simulink model "a2bcpwm_inverter_final"  (R2021b)
settings: Solver=VariableStepAuto  StartTime=0.0  StopTime=1.8  RelTol=1e-3
libraries: spsMosfetLib x8, spsSeriesRLCBranchLib x6, spsVoltageMeasurementLib x5, spsCurrentMeasurementLib x3, spsRMSLib x3, spsFourierLib x2, spsTriangleGeneratorLib x2, spsDCVoltageSourceLib x1, spsDiodeLib x1, spsMeanLib x1, spspowerguiLib x1
settings Model: Creator=adars  LastModifiedBy=basti
settings SolverCC: ZeroCrossAlgorithm=Adaptive
settings DebuggingCC: IgnoredZcDiagnostic=none  UnconnectedInputMsg=none  UnconnectedOutputMsg=none  UnconnectedLineMsg=none
settings ModelReferenceCC: EnableRefExpFcnMdlSchedulingChecks=off
settings RTWCC: DLArmComputeVersion=20.02.1

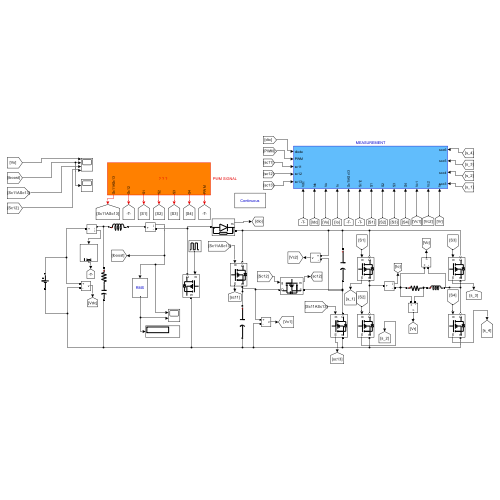
[thumbnail: Simulink's stored preview of the top-level diagram]
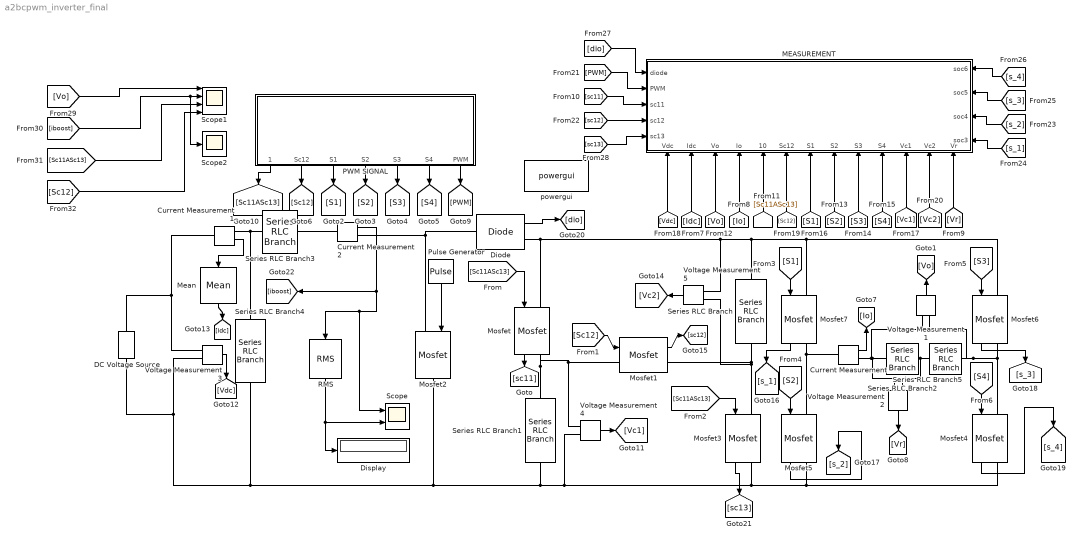
== system a2bcpwm_inverter_final ==
  Current Measurement : spsCurrentMeasurementLib/Current Measurement  PhasorSimulation=off  OutputType=Complex  PSBequivalent=0
  Current Measurement1 : spsCurrentMeasurementLib/Current Measurement  PhasorSimulation=off  OutputType=Complex  PSBequivalent=0
  Current Measurement2 : spsCurrentMeasurementLib/Current Measurement  PhasorSimulation=off  OutputType=Complex  PSBequivalent=0
  DC Voltage Source : spsDCVoltageSourceLib/DC Voltage Source  Amplitude=24  Measurements=None
  Diode : spsDiodeLib/Diode  Ron=0.001  Lon=0  Vf=0.8  IC=0  UseSnubber=0  Rs=500  Cs=250e-9  Measurements=on
  Display : Display
  MEASUREMENT : Subsystem
      settings: PortSchema="{\"entries\":[{\"content\":{\"sides\":[{\"content\":{\"connectorIds\":[\"In1\",\"In2\",\"In3\",\"In4\",\"In5\"]},\"type\":\"ConnectorPlacement.EquallySpacedRectSide\",\"uuid\":\"d6dfc44f-8fba-4c4a-86af-0984d0d1ef13\"},{\"content\":{\"connectorIds\":[\"In19\",\"In20\",\"In21\",\"In22\"],\"side\":\"RIGHT\"},\"type\":\"ConnectorPlacement.EquallySpacedRectSide\",\"uuid\":\"d6149925-38bb-4c16-a1b8-fa53fbdb5b8e\"},{\"content\":{\"connectorIds\":[],\"side\":\"TOP\"},\"type\":\"ConnectorPlacement.EquallySpacedRectSide\",\"uuid\":\"0a993214-5764-4564-a5db-9fa5a3117433\"},{\"content\":{\"connectorIds\":[\"In6\",\"In7\",\"In8\",\"In9\",\"In10\",\"In11\",\"In12\",\"In13\",\"In14\",\"In15\",\"In16\",\"In17\",\"In18\"],\"side\":\"BOTTOM\"},\"type\":\"ConnectorPlacement.EquallySpacedRectSide\",\"uuid\":\"ef2b73df-4ab0-44d0-8380-8491338002fd\"}]},\"type\":\"ConnectorPlacement.EquallySpacedConnector\",\"uuid\":\"c728dddf-1d1a-4ffc-a551-ed9f27d05892\"}],\"packageUris\":[\"http://schema.mathworks.com/mf0/Connector/R2020b\"],\"version\":\"1.0\"}"
  Mean : spsMeanLib/Mean  Freq=50  Vinit=0  Ts=0
  Mosfet{,1,3..7} (7 alike) : spsMosfetLib/Mosfet  Ron=0.1  Lon=0  Rd=0.01  Vfd=0  IC=0  Rs=1e5  Cs=inf  Measurements=on
  Mosfet2 : spsMosfetLib/Mosfet  Ron=0.1  Lon=0  Rd=0.01  Vfd=0  IC=0  Rs=1e5  Cs=inf  Measurements=off
  PWM SIGNAL : Subsystem
      mask Display: image('C:\Users\charl\Downloads\Screenshot 2023-01-03 005642.jpg'); % Use "Edit Image" on toolstrip to change.
  Pulse Generator : DiscretePulseGenerator  PulseType=Time based  Period=1/20000  PulseWidth=80
  RMS : spsRMSLib/RMS  TrueRMS=on  Freq=60  RMSInit=120  Ts=0
  Scope : Scope  NumInputPorts=2
  Scope1 : Scope  NumInputPorts=4
  Scope2 : Scope
  Series RLC Branch : spsSeriesRLCBranchLib/Series RLC Branch  LConnTagsString=__new0  RConnTagsString=__new0  BranchType=C  Resistance=1  Inductance=1e-3  SetiL0=off  InitialCurrent=0  Capacitance=3.9e-3  Setx0=off  InitialVoltage=0  Measurements=None
  Series RLC Branch1 : spsSeriesRLCBranchLib/Series RLC Branch  LConnTagsString=__new0  RConnTagsString=__new0  BranchType=C  Resistance=1  Inductance=1e-3  SetiL0=off  InitialCurrent=0  Capacitance=3.9e-3  Setx0=off  InitialVoltage=0  Measurements=None
  Series RLC Branch2 : spsSeriesRLCBranchLib/Series RLC Branch  LConnTagsString=__new0  RConnTagsString=__new0  BranchType=R  Resistance=70  Inductance=150e-3  SetiL0=off  InitialCurrent=0  Capacitance=1e-6  Setx0=off  InitialVoltage=0  Measurements=None
  Series RLC Branch3 : spsSeriesRLCBranchLib/Series RLC Branch  LConnTagsString=__new0  RConnTagsString=__new0  BranchType=L  Resistance=1.5  Inductance=0.9e-3  SetiL0=off  InitialCurrent=0  Capacitance=1e-6  Setx0=off  InitialVoltage=0  Measurements=None
  Series RLC Branch4 : spsSeriesRLCBranchLib/Series RLC Branch  LConnTagsString=__new0  RConnTagsString=__new0  BranchType=RC  Resistance=.0001  Inductance=1e-3  SetiL0=off  InitialCurrent=0  Capacitance=1e-3  Setx0=off  InitialVoltage=0  Measurements=None
  Series RLC Branch5 : spsSeriesRLCBranchLib/Series RLC Branch  LConnTagsString=__new0  RConnTagsString=__new0  BranchType=L  Resistance=100  Inductance=.129  SetiL0=off  InitialCurrent=0  Capacitance=1e-6  Setx0=off  InitialVoltage=0  Measurements=None
  Voltage Measurement{1..5} (5 alike) : spsVoltageMeasurementLib/Voltage Measurement  PhasorSimulation=off  OutputType=Complex  PSBequivalent=0
  powergui : spspowerguiLib/powergui  Priority=1  SimulationMode=Continuous  SampleTime=50e-6  frequency=60  Iterations=50  frequencyindice=0  Pbase=100e6  ErrMax=1e-4  UnitsV=kV  UnitsW=MW  buscounter=0  FunctionMessages=off  echomessages=off  EnableUseOfTLC=off  CurrentSourceSwitches=off  DisableSnubberDevices=off  DisableRonSwitches=off  DisableVfSwitches=off  DisplayEquations=off  AutomaticDiscreteSolvers=off  SolverType=Tustin/Backward Euler (TBE)  Interpol=off  ExternalGateDelay=off  methode=off  Ts=100  x0status=blocks  SPID=on  SwTol=0  HookPort=off  NonlinearTolerance=1e-4  nMaxIteration=100  ContinueOnMaxIteration=off  RestoreLinks=warning  ResistiveCurrentMeasurement=off  Frange=[0:2:500]  Ylog=off  Xlog=on  ShowGrid=off  save=off  variable=ZData  structure=0  ZoomFFT=off  StartTime=0.0  cycles=1  DisplayStyle=1  fundamental=60  FreqAxis=off  MaxFrequency=1000  frequencyindicesteady=1  RmsSteady=1  display=off
  wires:
  PWM SIGNAL/1(Sc11ASc13) -> [Sc11ASc13]
  PWM SIGNAL/6(S4) -> [S4]
  PWM SIGNAL/5(S3) -> [S3]
  PWM SIGNAL/3(S1) -> [S1]
  PWM SIGNAL/2(Sc12) -> [Sc12]
  [Sc11ASc13] -> Mosfet/1
  [Sc12] -> Mosfet1/1
  [Sc11ASc13] -> Mosfet3/1
  [S1] -> Mosfet7/1
  [S2] -> Mosfet5/1
  [S3] -> Mosfet6/1
  [S4] -> Mosfet4/1
  PWM SIGNAL/4(S2) -> [S2]
  Current Measurement/1 -> [Io]
  [Vo] -> MEASUREMENT/8(Vo)
  [Io] -> MEASUREMENT/9(Io)
  [Sc11ASc13] -> MEASUREMENT/10(Sc11ASc13)
  [Sc12] -> MEASUREMENT/11(Sc12)
  [S1] -> MEASUREMENT/12(S1)
  [S2] -> MEASUREMENT/13(S2)
  [S3] -> MEASUREMENT/14(S3)
  [S4] -> MEASUREMENT/15(S4)
  PWM SIGNAL/7(PWM) -> [PWM]
  Pulse Generator/1 -> Mosfet2/1
  Voltage Measurement1/1 -> [Vo]
  [Idc] -> MEASUREMENT/7(Idc)
  Voltage Measurement3/1 -> [Vdc]
  [Vdc] -> MEASUREMENT/6(Vdc)
  Voltage Measurement4/1 -> [Vc1]
  Voltage Measurement5/1 -> [Vc2]
  Current Measurement1/1 -> Mean/1
  Mean/1 -> [Idc]
  [Vc1] -> MEASUREMENT/16(Vc1)
  [Vc2] -> MEASUREMENT/17(Vc2)
  [PWM] -> MEASUREMENT/2(PWM)
  Voltage Measurement2/1 -> [Vr]
  [Vr] -> MEASUREMENT/18(Vr)
  Mosfet/1 -> [sc11]
  Mosfet1/1 -> [sc12]
  [sc12] -> MEASUREMENT/4(sc12)
  [sc11] -> MEASUREMENT/3(sc11)
  Mosfet7/1 -> [s_1]
  Mosfet5/1 -> [s_2]
  Mosfet6/1 -> [s_3]
  Mosfet4/1 -> [s_4]
  [s_2] -> MEASUREMENT/21(soc4)
  [s_1] -> MEASUREMENT/22(soc3)
  [s_3] -> MEASUREMENT/20(soc5)
  [s_4] -> MEASUREMENT/19(soc6)
  Diode/1 -> [dio]
  [dio] -> MEASUREMENT/1(diode)
  Mosfet3/1 -> [sc13]
  [sc13] -> MEASUREMENT/5(sc13)
  Current Measurement2/1 -> [iboost], Scope/1, RMS/1
  RMS/1 -> Display/1, Scope/2
  [Vo] -> Scope1/1
  [iboost] -> Scope2/1, Scope1/2
  [Sc11ASc13] -> Scope1/3
  [Sc12] -> Scope1/4
  connections:
  Mosfet4/LConn1 -- Voltage Measurement1/LConn2 -- Series RLC Branch5/RConn1 -- Mosfet6/RConn1
  Series RLC Branch2/LConn1 -- Current Measurement/RConn1 -- Voltage Measurement1/LConn1 -- Voltage Measurement2/LConn1
  Series RLC Branch/RConn1 -- Mosfet3/LConn1 -- Voltage Measurement5/LConn2 -- Mosfet1/RConn1
  Mosfet/RConn1 -- Voltage Measurement4/LConn1 -- Mosfet1/LConn1 -- Series RLC Branch1/LConn1
  Mosfet7/LConn1 -- Voltage Measurement5/LConn1 -- Mosfet/LConn1 -- Diode/RConn1 -- Series RLC Branch/LConn1 -- Mosfet6/LConn1
  Mosfet7/RConn1 -- Mosfet5/LConn1 -- Current Measurement/LConn1
  Series RLC Branch4/LConn1 -- Current Measurement1/RConn1 -- Series RLC Branch3/LConn1
  Mosfet5/RConn1 -- Voltage Measurement4/LConn2 -- Series RLC Branch1/RConn1 -- DC Voltage Source/LConn1 -- Voltage Measurement3/LConn2 -- Series RLC Branch4/RConn1 -- Mosfet2/RConn1 -- Mosfet3/RConn1 -- Mosfet4/RConn1
  Voltage Measurement3/LConn1 -- DC Voltage Source/RConn1 -- Current Measurement1/LConn1
  Voltage Measurement2/LConn2 -- Series RLC Branch2/RConn1 -- Series RLC Branch5/LConn1
  Mosfet2/LConn1 -- Current Measurement2/RConn1 -- Diode/LConn1
  Current Measurement2/LConn1 -- Series RLC Branch3/RConn1

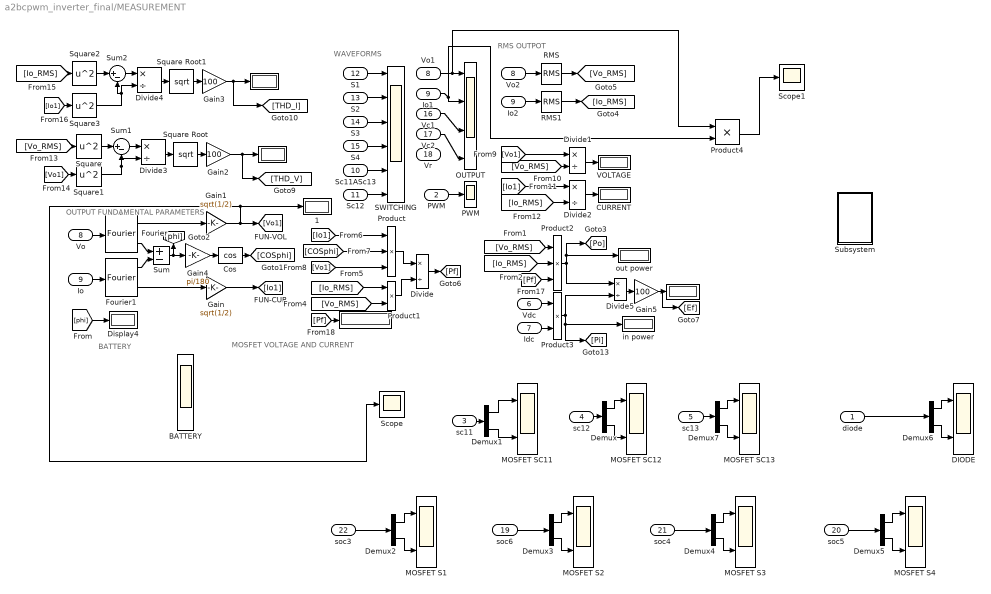
== system a2bcpwm_inverter_final/MEASUREMENT ==
  note: MOSFET VOLTAGE AND
      | CURRENT
  note: BATTERY
  note: WAVEFORMS
  note: OUTPUT FUNDAMENTAL PARAMETERS
  note: RMS OUTPOT
  diode : Inport
  PWM : Inport  Port=2
  sc11 : Inport  Port=3
  sc12 : Inport  Port=4
  sc13 : Inport  Port=5
  Vdc : Inport  Port=6
  Idc : Inport  Port=7
  Vo : Inport  Port=8
  Io : Inport  Port=9
  Sc11ASc13 : Inport  Port=10
  Sc12 : Inport  Port=11
  S1 : Inport  Port=12
  S2 : Inport  Port=13
  S3 : Inport  Port=14
  S4 : Inport  Port=15
  Vc1 : Inport  Port=16
  Vc2 : Inport  Port=17
  Vr : Inport  Port=18
  soc6 : Inport  Port=19
  soc5 : Inport  Port=20
  soc4 : Inport  Port=21
  soc3 : Inport  Port=22
  " " : Display
  "  " : Display
  "   " : Display
  "        " : Display
  "   1" : Display
  "  VOLTAGE  " : Display
  " out power" : Display
  BATTERY : Scope  NumInputPorts=3
  CURRENT : Display
  Cos : Trigonometry  Operator=cos
  DIODE : Scope  NumInputPorts=2
  Demux{,1..7} (8 alike) : Demux  Outputs=2
  Display4 : Display
  Divide{,1..5} (6 alike) : Product  Inputs=*/
  Fourier : spsFourierLib/Fourier  Freq=50  n=1  InInit=[0, 0]  Ts=0
  Fourier1 : spsFourierLib/Fourier  Freq=50  n=1  InInit=[0, 0]  Ts=0
  Gain : Gain  Gain=sqrt(1/2)
  Gain1 : Gain  Gain=sqrt(1/2)
  Gain2 : Gain  Gain=100
  Gain3 : Gain  Gain=100
  Gain4 : Gain  Gain=pi/180
  Gain5 : Gain  Gain=100
  Io1 : InportShadow  Port=9
  Io2 : InportShadow  Port=9
  MOSFET S{1..4} (4 alike) : Scope  NumInputPorts=2
  MOSFET SC11 : Scope  NumInputPorts=2
  MOSFET SC12 : Scope  NumInputPorts=2
  MOSFET SC13 : Scope  NumInputPorts=2
  OUTPUT : Scope  NumInputPorts=4
  "PWM " : Scope
  Product : Product  Inputs=3
  Product1 : Product
  Product2 : Product  Inputs=***
  Product3 : Product  Inputs=**
  Product4 : Product
  RMS : spsRMSLib/RMS  TrueRMS=on  Freq=50  RMSInit=120  Ts=0
  RMS1 : spsRMSLib/RMS  TrueRMS=on  Freq=50  RMSInit=120  Ts=0
  SWITCHING : Scope  NumInputPorts=6
  Scope : Scope
  Scope1 : Scope
  Square{,1..3} (4 alike) : Math  Operator=square  SaturateOnIntegerOverflow=on
  Square Root : Sqrt  SaturateOnIntegerOverflow=on
  Square Root1 : Sqrt  SaturateOnIntegerOverflow=on
  Subsystem : Subsystem
  Sum : Sum  Inputs=+-
  Sum1 : Sum  Inputs=|+-
  Sum2 : Sum  Inputs=|+-
  Vo1 : InportShadow  Port=8
  Vo2 : InportShadow  Port=8
  in power : Display
  wires:
  Sc11ASc13/1 -> SWITCHING/5
  Sc12/1 -> SWITCHING/6
  S1/1 -> SWITCHING/1
  S2/1 -> SWITCHING/2
  S3/1 -> SWITCHING/3
  S4/1 -> SWITCHING/4
  Vo/1 -> Fourier/1
  Io/1 -> Fourier1/1
  Fourier/1 -> Gain1/1
  Fourier/2 -> Sum/1
  Fourier1/1 -> Gain/1
  Fourier1/2 -> Sum/2
  Sum/1 -> Gain4/1, [phi]
  Gain/1 -> [Io1]
  Gain1/1 -> "   1"/1, Scope/1, [Vo1]
  Vo2/1 -> RMS/1
  Io2/1 -> RMS1/1
  RMS1/1 -> [Io_RMS]
  Cos/1 -> [COSphi]
  Product/1 -> Divide/1
  Product1/1 -> Divide/2
  Divide/1 -> [Pf]
  RMS/1 -> [Vo_RMS]
  [Io1] -> Product/1
  [Vo1] -> Product/3
  [COSphi] -> Product/2
  [Io_RMS] -> Product1/1
  [Vo_RMS] -> Product1/2
  [Vo1] -> Divide1/1
  [Vo_RMS] -> Divide1/2
  [Io1] -> Divide2/1
  [Io_RMS] -> Divide2/2
  Divide1/1 -> "  VOLTAGE  "/1
  Divide2/1 -> CURRENT/1
  [Vo_RMS] -> Square/1
  [Vo1] -> Square1/1
  Square/1 -> Sum1/1
  Square1/1 -> Divide3/2, Sum1/2
  Sum1/1 -> Divide3/1
  Divide3/1 -> Square Root/1
  Square2/1 -> Sum2/1
  Sum2/1 -> Divide4/1
  [Io_RMS] -> Square2/1
  [Io1] -> Square3/1
  Square3/1 -> Divide4/2, Sum2/2
  Divide4/1 -> Square Root1/1
  [phi] -> Display4/1
  [Vo_RMS] -> Product2/1
  [Io_RMS] -> Product2/2
  [Pf] -> Product2/3
  Vdc/1 -> Product3/1
  Idc/1 -> Product3/2
  Square Root/1 -> Gain2/1
  Square Root1/1 -> Gain3/1
  Gain4/1 -> Cos/1
  [Pf] -> "        "/1
  Vo1/1 -> Product4/1, OUTPUT/1
  Vc1/1 -> OUTPUT/3
  PWM/1 -> "PWM "/1
  Vc2/1 -> OUTPUT/4
  Io1/1 -> Product4/2, OUTPUT/2
  Divide5/1 -> Gain5/1
  sc12/1 -> Demux/1
  Demux/1 -> MOSFET SC12/1
  Demux/2 -> MOSFET SC12/2
  Demux1/1 -> MOSFET SC11/1
  sc11/1 -> Demux1/1
  Demux1/2 -> MOSFET SC11/2
  Gain2/1 -> "  "/1, [THD_V]
  Gain3/1 -> "   "/1, [THD_I]
  Product3/1 -> [Pi], in power/1, Divide5/2
  Product2/1 -> [Po], " out power"/1, Divide5/1
  Gain5/1 -> [Ef], " "/1
  Demux4/1 -> MOSFET S3/1
  Demux3/2 -> MOSFET S2/2
  soc4/1 -> Demux4/1
  soc6/1 -> Demux3/1
  Demux3/1 -> MOSFET S2/1
  soc5/1 -> Demux5/1
  Demux4/2 -> MOSFET S3/2
  Demux5/1 -> MOSFET S4/1
  Demux5/2 -> MOSFET S4/2
  diode/1 -> Demux6/1
  Demux6/1 -> DIODE/1
  Demux6/2 -> DIODE/2
  Demux7/2 -> MOSFET SC13/2
  Demux7/1 -> MOSFET SC13/1
  sc13/1 -> Demux7/1
  Demux2/2 -> MOSFET S1/2
  Demux2/1 -> MOSFET S1/1
  soc3/1 -> Demux2/1
  Product4/1 -> Scope1/1

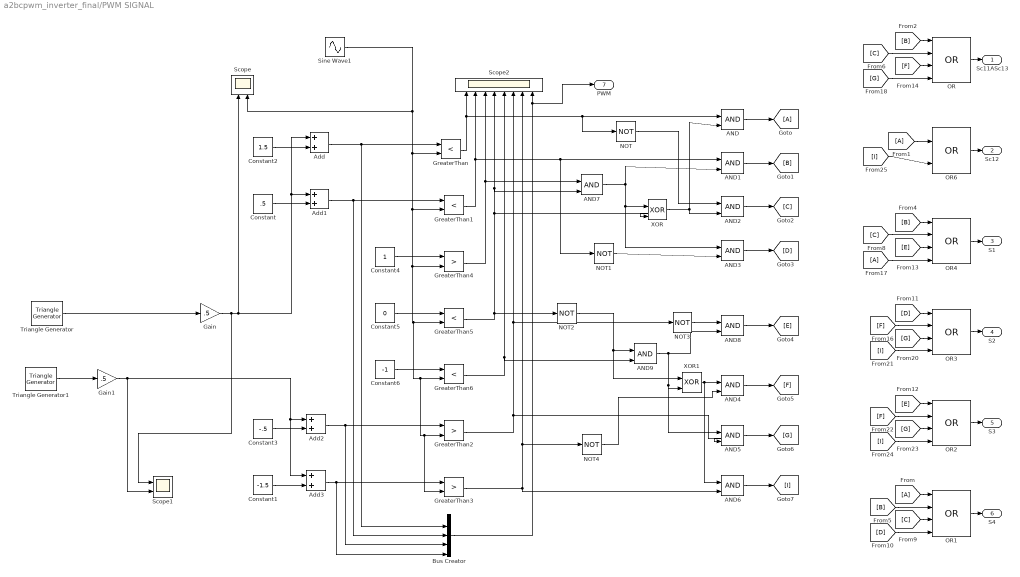
== system a2bcpwm_inverter_final/PWM SIGNAL ==
  AND{,1..9} (10 alike) : Logic  IconShape=distinctive  AllPortsSameDT=off  OutDataTypeStr=boolean
  Add{,1..3} (4 alike) : Sum
  Bus Creator : BusCreator  Inputs=5
  Constant : Constant  Value=.5
  Constant1 : Constant  Value=-1.5
  Constant2 : Constant  Value=1.5
  Constant3 : Constant  Value=-.5
  Constant4 : Constant
  Constant5 : Constant  Value=0
  Constant6 : Constant  Value=-1
  Gain : Gain  Gain=.5
  Gain1 : Gain  Gain=.5
  GreaterThan{,1,5..6} (4 alike) : RelationalOperator  Operator=<  OutDataTypeStr=boolean  RndMeth=Simplest
  GreaterThan2 : RelationalOperator  Operator=>  OutDataTypeStr=boolean  RndMeth=Simplest
  GreaterThan3 : RelationalOperator  Operator=>  OutDataTypeStr=boolean  RndMeth=Simplest
  GreaterThan4 : RelationalOperator  Operator=>  OutDataTypeStr=boolean  RndMeth=Simplest
  NOT{,1..4} (5 alike) : Logic  Operator=NOT  IconShape=distinctive  AllPortsSameDT=off  OutDataTypeStr=boolean
  OR{,1..4} (5 alike) : Logic  Operator=OR  Inputs=4  IconShape=distinctive  AllPortsSameDT=off  OutDataTypeStr=boolean
  OR6 : Logic  Operator=OR  IconShape=distinctive  AllPortsSameDT=off  OutDataTypeStr=boolean
  Scope : Scope  NumInputPorts=2
  Scope1 : Scope  NumInputPorts=2
  Scope2 : Scope  NumInputPorts=8
  Sine Wave1 : Sin  Amplitude=1.9  Frequency=50*2*pi  SampleTime=0
  Triangle Generator : spsTriangleGeneratorLib/Triangle Generator  Freq=20000  Phase=0  Ts=0
  Triangle Generator1 : spsTriangleGeneratorLib/Triangle Generator  Freq=20000  Phase=180  Ts=0
  XOR : Logic  Operator=XOR  IconShape=distinctive  AllPortsSameDT=off  OutDataTypeStr=boolean
  XOR1 : Logic  Operator=XOR  IconShape=distinctive  AllPortsSameDT=off  OutDataTypeStr=boolean
  Sc11ASc13 : Outport
  Sc12 : Outport  Port=2
  S1 : Outport  Port=3
  S2 : Outport  Port=4
  S3 : Outport  Port=5
  S4 : Outport  Port=6
  PWM : Outport  Port=7
  wires:
  GreaterThan3/1 -> Scope2/7, NOT4/1, AND6/2
  GreaterThan4/1 -> Scope2/3, AND7/1
  [F] -> OR/3
  GreaterThan5/1 -> XOR/2, AND7/2, Scope2/4, NOT2/1
  AND8/1 -> [E]
  Add/1 -> GreaterThan/1, Bus Creator/2
  Constant/1 -> Add1/2
  NOT4/1 -> AND4/2
  AND3/1 -> [D]
  AND1/1 -> [B]
  GreaterThan1/1 -> NOT1/1, AND1/1, Scope2/2
  Constant6/1 -> GreaterThan6/1
  [E] -> OR2/1
  [D] -> OR3/1
  AND9/1 -> AND8/2, XOR1/2, AND5/1
  [C] -> OR/2
  [G] -> OR2/3
  OR/1 -> Sc11ASc13/1
  [I] -> OR6/2
  OR2/1 -> S3/1
  [B] -> OR4/1
  [C] -> OR4/2
  OR3/1 -> S2/1
  Add2/1 -> Bus Creator/4, GreaterThan2/1
  Constant3/1 -> Add2/2
  AND7/1 -> XOR/1, AND3/1, AND1/2
  AND6/1 -> [I]
  NOT/1 -> AND2/1
  XOR1/1 -> AND6/1, AND4/1
  Constant4/1 -> GreaterThan4/1
  [G] -> OR/4
  [I] -> OR2/4
  NOT2/1 -> AND9/1, XOR1/1
  Constant1/1 -> Add3/2
  [A] -> OR1/1
  AND4/1 -> [F]
  [B] -> OR/1
  NOT1/1 -> AND3/2
  Add3/1 -> Bus Creator/5, GreaterThan3/1
  GreaterThan/1 -> AND/1, NOT/1, Scope2/1
  [A] -> OR6/1
  AND2/1 -> [C]
  [F] -> OR2/2
  Add1/1 -> GreaterThan1/1, Bus Creator/3
  AND/1 -> [A]
  [B] -> OR1/2
  Constant5/1 -> GreaterThan5/1
  [I] -> OR3/4
  [F] -> OR3/2
  GreaterThan6/1 -> AND9/2, Scope2/5
  Bus Creator/1 -> PWM/1, Scope2/8
  GreaterThan2/1 -> Scope2/6, NOT3/1, AND5/2
  Constant2/1 -> Add/2
  NOT3/1 -> AND8/1
  XOR/1 -> AND/2, AND2/2
  AND5/1 -> [G]
  [D] -> OR1/4
  [C] -> OR1/3
  [A] -> OR4/4
  [E] -> OR4/3
  [G] -> OR3/3
  OR4/1 -> S1/1
  OR1/1 -> S4/1
  OR6/1 -> Sc12/1
  Triangle Generator/1 -> Gain/1
  Gain/1 -> Scope1/1, Scope/1, Add/1, Add1/1
  Sine Wave1/1 -> Scope/2, GreaterThan1/2, GreaterThan4/2, GreaterThan3/2, GreaterThan2/2, GreaterThan6/2, GreaterThan5/2, GreaterThan/2
  Triangle Generator1/1 -> Gain1/1
  Gain1/1 -> Add3/1, Add2/1, Scope1/2

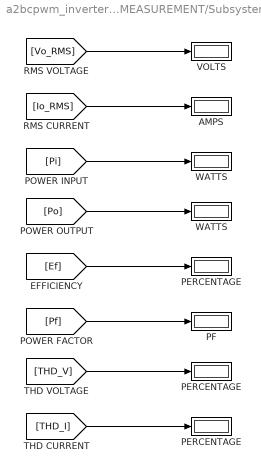
== system a2bcpwm_inverter_final/MEASUREMENT/Subsystem ==
  "  PERCENTAGE" : Display
  " PERCENTAGE" : Display
  " PERCENTAGE " : Display
  " PF" : Display
  " VOLTS" : Display
  " WATTS" : Display
  " WATTS " : Display
  AMPS : Display
  wires:
  [THD_V] -> " PERCENTAGE "/1
  [Pf] -> " PF"/1
  [THD_I] -> "  PERCENTAGE"/1
  [Po] -> " WATTS "/1
  [Vo_RMS] -> " VOLTS"/1
  [Ef] -> " PERCENTAGE"/1
  [Pi] -> " WATTS"/1
  [Io_RMS] -> AMPS/1
